simulink model "SimuLinkD2SL"  (R2025b)
settings: Solver=ode4  StartTime=0.0  StopTime=110  FixedStep=1e-3  RelTol=1e-3
settings Model: Creator=luketucker  LastModifiedBy=luketucker

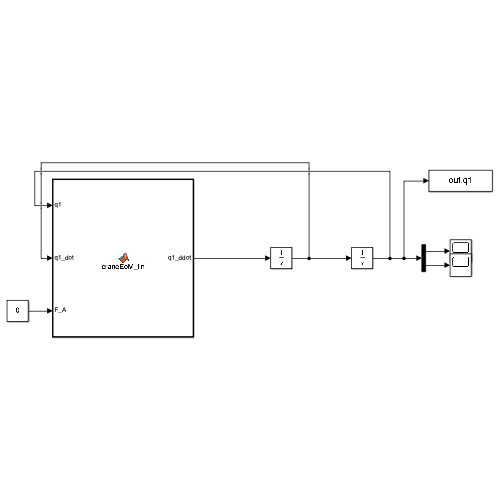
[thumbnail: Simulink's stored preview of the top-level diagram]
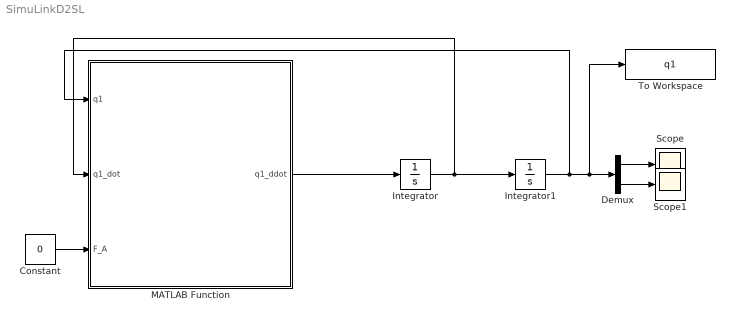
== system SimuLinkD2SL ==
  Constant : Constant  Value=0
  Demux : Demux  Outputs=2
  Integrator : Integrator  InitialCondition=[0;0]
  Integrator1 : Integrator  InitialCondition=[11.5;pi/3]
  MATLAB Function : MATLAB Function  TreatAsAtomicUnit=on
  Scope : Scope
      settings: ActiveDisplayYMinimum=-1  ActiveDisplayYMaximum=1
  Scope1 : Scope
      settings: ActiveDisplayYMinimum=-1  ActiveDisplayYMaximum=1
  To Workspace : ToWorkspace  VariableName=q1  SampleTime=-1
  wires:
  MATLAB Function/1(q1_ddot) -> Integrator/1
  Integrator/1 -> Integrator1/1, MATLAB Function/2(q1_dot)
  Integrator1/1 -> To Workspace/1, Demux/1, MATLAB Function/1(q1)
  Constant/1 -> MATLAB Function/3(F_A)
  Demux/1 -> Scope/1
  Demux/2 -> Scope1/1

== matlab function SimuLinkD2SL/MATLAB Function ==
  data: q1 input; q1_ddot output; q1_dot input; F_A input
function q1_ddot = craneEoM_lin(q1, q1_dot, F_A)




    %Generalized coordinates
    x1          = q1(1);
    theta1      = q1(2);
    x1_dot      = q1_dot(1);
    theta1_dot  = q1_dot(2);


    M = craneM_lin_sym( x1, theta1, x1_dot, theta1_dot, F_A );
    F = craneF_lin_sym( x1, theta1, x1_dot, theta1_dot, F_A );

    % Solve for accelerations
    q1_ddot = M \ F;     % 2x1: [x_ddot; theta_ddot]


end
